simulink model "Speed_Limiter"  (R2022b)
settings: configuration reference "CommonModelConfiguration" (kept outside this file)
undefined symbols (not defined in the file): cc_param_36, LCFG_ActivationDeactivation, LCFG_DSF_Timeout, LCFG_SL_IntStsDelay, LCFG_SL_Tmr1, LCFG_SL_Tmr2
settings Model: Creator=rkallum  LastModifiedBy=OTHOMSO1
settings ConfigSetRef: SourceName=CommonModelConfiguration  SourceLocation=Base Workspace

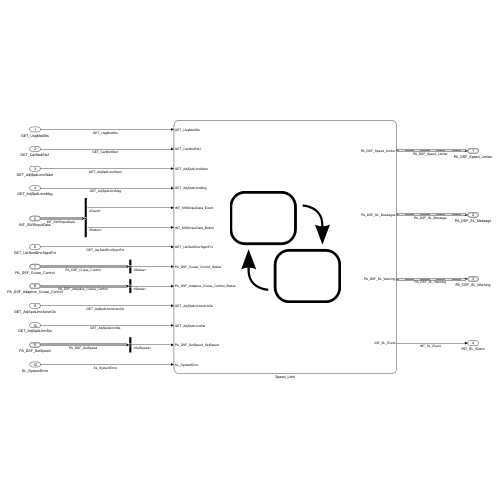
[thumbnail: Simulink's stored preview of the top-level diagram]
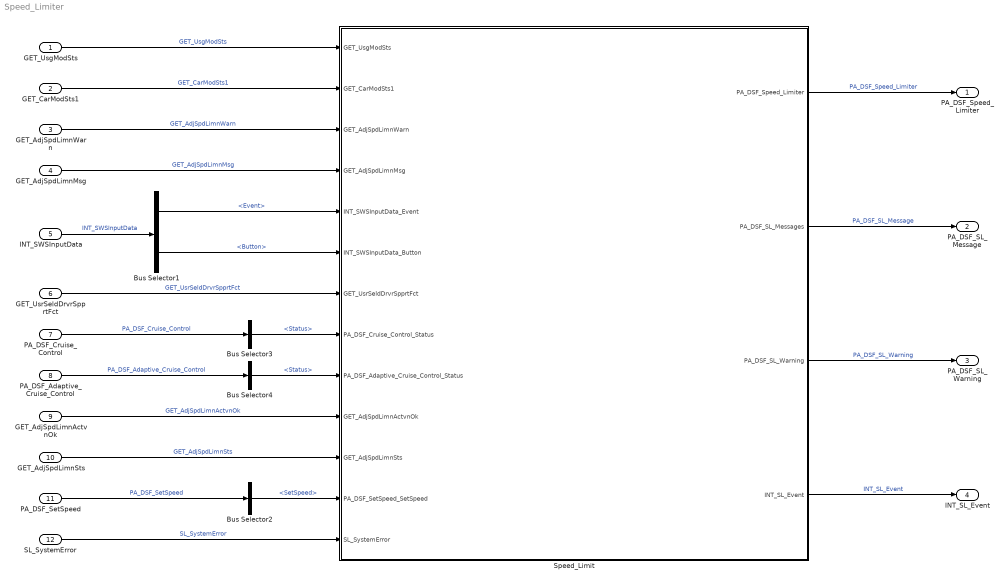
== system Speed_Limiter ==
  GET_UsgModSts : Inport
  GET_CarModSts1 : Inport  Port=2
  GET_AdjSpdLimnWarn : Inport  Port=3
  GET_AdjSpdLimnMsg : Inport  Port=4
  INT_SWSInputData : Inport  Port=5  OutDataTypeStr=Bus: SWSInputData  LockScale=on
  GET_UsrSeldDrvrSpprtFct : Inport  Port=6
  PA_DSF_Cruise_Control : Inport  Port=7  OutDataTypeStr=Bus: PA_DSF
  PA_DSF_Adaptive_Cruise_Control : Inport  Port=8  OutDataTypeStr=Bus: PA_DSF_ACC
  GET_AdjSpdLimnActvnOk : Inport  Port=9
  GET_AdjSpdLimnSts : Inport  Port=10
  PA_DSF_SetSpeed : Inport  Port=11  OutDataTypeStr=Bus: PA_StatusAndValueAndDoubleAndDouble
  SL_SystemError : Inport  Port=12  OutDataTypeStr=boolean
  Bus Selector1 : BusSelector  OutputSignals=Event,Button
  Bus Selector2 : BusSelector  OutputSignals=SetSpeed
  Bus Selector3 : BusSelector  OutputSignals=Status
  Bus Selector4 : BusSelector  OutputSignals=Status
  Speed_Limit : Stateflow chart  TreatAsAtomicUnit=on
  PA_DSF_Speed_Limiter : Outport  OutDataTypeStr=Bus: PA_DSF  VectorParamsAs1DForOutWhenUnconnected=off
  PA_DSF_SL_Message : Outport  Port=2  OutDataTypeStr=Bus: PA_DSF_Message  VectorParamsAs1DForOutWhenUnconnected=off
  PA_DSF_SL_Warning : Outport  Port=3  OutDataTypeStr=Bus: PA_StatusAndOffOnValue  VectorParamsAs1DForOutWhenUnconnected=off
  INT_SL_Event : Outport  Port=4  OutDataTypeStr=Enum: E_DSF_Event  VectorParamsAs1DForOutWhenUnconnected=off
  wires:
  Speed_Limit/1(PA_DSF_Speed_Limiter) -> PA_DSF_Speed_Limiter/1  "PA_DSF_Speed_Limiter"
  Speed_Limit/2(PA_DSF_SL_Messages) -> PA_DSF_SL_Message/1  "PA_DSF_SL_Message"
  Speed_Limit/3(PA_DSF_SL_Warning) -> PA_DSF_SL_Warning/1  "PA_DSF_SL_Warning"
  Speed_Limit/4(INT_SL_Event) -> INT_SL_Event/1  "INT_SL_Event"
  GET_CarModSts1/1 -> Speed_Limit/2(GET_CarModSts1)  "GET_CarModSts1"
  GET_AdjSpdLimnWarn/1 -> Speed_Limit/3(GET_AdjSpdLimnWarn)  "GET_AdjSpdLimnWarn"
  GET_AdjSpdLimnMsg/1 -> Speed_Limit/4(GET_AdjSpdLimnMsg)  "GET_AdjSpdLimnMsg"
  GET_UsrSeldDrvrSpprtFct/1 -> Speed_Limit/7(GET_UsrSeldDrvrSpprtFct)  "GET_UsrSeldDrvrSpprtFct"
  GET_AdjSpdLimnActvnOk/1 -> Speed_Limit/10(GET_AdjSpdLimnActvnOk)  "GET_AdjSpdLimnActvnOk"
  GET_AdjSpdLimnSts/1 -> Speed_Limit/11(GET_AdjSpdLimnSts)  "GET_AdjSpdLimnSts"
  GET_UsgModSts/1 -> Speed_Limit/1(GET_UsgModSts)  "GET_UsgModSts"
  PA_DSF_Cruise_Control/1 -> Bus Selector3/1  "PA_DSF_Cruise_Control"
  PA_DSF_Adaptive_Cruise_Control/1 -> Bus Selector4/1  "PA_DSF_Adaptive_Cruise_Control"
  PA_DSF_SetSpeed/1 -> Bus Selector2/1  "PA_DSF_SetSpeed"
  SL_SystemError/1 -> Speed_Limit/13(SL_SystemError)  "SL_SystemError"
  INT_SWSInputData/1 -> Bus Selector1/1  "INT_SWSInputData"
  Bus Selector1/1 -> Speed_Limit/5(INT_SWSInputData_Event)  "<Event>"
  Bus Selector1/2 -> Speed_Limit/6(INT_SWSInputData_Button)  "<Button>"
  Bus Selector2/1 -> Speed_Limit/12(PA_DSF_SetSpeed_SetSpeed)  "<SetSpeed>"
  Bus Selector3/1 -> Speed_Limit/8(PA_DSF_Cruise_Control_Status)  "<Status>"
  Bus Selector4/1 -> Speed_Limit/9(PA_DSF_Adaptive_Cruise_Control_Status)  "<Status>"

== stateflow chart Speed_Limiter/Speed_Limit ==
  state CARCONFIG_INVALID
    entry:  PA_DSF_Speed_Limiter.Status=E_CommonStatus.NotPresent;
    PA_DSF_SL_Messages.Status=E_CommonStatus.NotPresent;
    PA_DSF_SL_Warning.Status=E_CommonStatus.NotPresent;
    PA_DSF_Speed_Limiter.Value=E_DSF_Value.DSF_Selected;
    PA_DSF_SL_Warning.Value=E_OffOn.Off;
    INT_SL_Event=E_DSF_Event.NoReq;
  state SYSTEM_OK
    state NOT_ACTIVE
      entry: PA_DSF_Speed_Limiter.Status=E_CommonStatus.Disabled;
      PA_DSF_SL_Messages.Status=E_CommonStatus.Disabled;
      PA_DSF_SL_Warning.Status=E_CommonStatus.Disabled;
      PA_DSF_SL_Warning.Value=E_OffOn.Off;
      INT_SL_Event=E_DSF_Event.NoReq;
      state MESSAGES_OFF
        entry:
        PA_DSF_SL_Messages.Value=E_DSF_Messages.Messages_Off;
        PA_DSF_Speed_Limiter.Value=E_DSF_Value.DSF_Selected;
      state CANCEL_WARNING
        entry:
        PA_DSF_SL_Messages.Value=E_DSF_Messages.Messages_CancelWarning;
        PA_DSF_Speed_Limiter.Value=E_DSF_Value.DSF_Selected;
      (default) -> (junction 220)
      (junction 220) -> (junction 224) [order 1] : [PA_DSF_Speed_Limiter.Value==E_DSF_Value.DSF_Active]
      (junction 220) -> MESSAGES_OFF [order 2]
      (junction 224) -> SYSTEM_OK.NOT_ACTIVE.CANCEL_WARNING
      SYSTEM_OK.NOT_ACTIVE.CANCEL_WARNING -> MESSAGES_OFF : [after(LCFG_DSF_Timeout, sec)]
    state PENDING
    state PENDING1
    state ACTIVE
      state WARNING [parallel]
        entry: PA_DSF_SL_Warning.Status=E_CommonStatus.Available;
        settings: executionOrder=1
        state ON
          entry: PA_DSF_SL_Warning.Value=E_OffOn.On;
        state OFF
          entry: PA_DSF_SL_Warning.Value=E_OffOn.Off;
        (default) -> OFF
        OFF -> SYSTEM_OK.ACTIVE.WARNING.ON : [PA_DSF_Speed_Limiter.Value==E_DSF_Value.DSF_Active &&...
            | (GET_AdjSpdLimnWarn==AdjSpdLimnWarnCoding.AdjSpdLimnWarnCoding_VisWarn ||...
            | GET_AdjSpdLimnWarn==AdjSpdLimnWarnCoding.AdjSpdLimnWarnCoding_SoundAndVisWarn)]
        SYSTEM_OK.ACTIVE.WARNING.ON -> OFF : [PA_DSF_Speed_Limiter.Value~=E_DSF_Value.DSF_Active ||...
            | (GET_AdjSpdLimnWarn~=AdjSpdLimnWarnCoding.AdjSpdLimnWarnCoding_VisWarn &&...
            | GET_AdjSpdLimnWarn~=AdjSpdLimnWarnCoding.AdjSpdLimnWarnCoding_SoundAndVisWarn)]
      state MESSAGES [parallel]
        entry: PA_DSF_SL_Messages.Status=E_CommonStatus.Available;
        settings: executionOrder=2
        state retVal = slMessages [function]
          state retVal2 = slActivationReq [function]
            (default) -> (junction 357)
            (junction 357) -> (junction 358) [order 1] : [(GET_AdjSpdLimnSts~=AdjSpdLimnSts2.AdjSpdLimnSts2_Actv)...
                | && (GET_AdjSpdLimnActvnOk == OnOff1.OnOff1_Off)...
                | && (INT_SWSInputData_Button ==  E_SWSButton.BtnL1Req)...
                | && (INT_SWSInputData_Event ==  E_SWSEvent.Push)]
            (junction 357) -> (junction 360) [order 2]
            (junction 358) -> (junction 359)
            (junction 360) -> (junction 359) [order 1] : [(GET_AdjSpdLimnSts~=AdjSpdLimnSts2.AdjSpdLimnSts2_Actv)...
                | && (GET_AdjSpdLimnActvnOk == OnOff1.OnOff1_Off)...
                | && (INT_SWSInputData_Button ==  E_SWSButton.BtnL5Req)...
                | && (INT_SWSInputData_Event ==  E_SWSEvent.Push)...
                | && (PA_DSF_SetSpeed_SetSpeed~=0)]
            (junction 359) -> (junction 361) : {retVal2 = true;}
            (junction 360) -> (junction 362) [order 2] : {retVal2 = false;}
            (junction 361) -> (junction 362)
            (junction 362) -> (junction 363)
          (default) -> (junction 391)
          (junction 391) -> (junction 374) [order 1] : [hasChangedTo(GET_AdjSpdLimnMsg,  AdjSpdLimnMsg1.AdjSpdLimnMsg1_AdjSpdLimnCncl)]
              | {PA_DSF_SL_Messages.Value=E_DSF_Messages.Messages_CancelWarning;}
          (junction 391) -> (junction 392) [order 2]
          (junction 374) -> (junction 375)
          (junction 392) -> (junction 375) [order 1] : [(GET_AdjSpdLimnMsg == AdjSpdLimnMsg1.AdjSpdLimnMsg1_AdjSpdLimnInhb) &&...
              | slActivationReq()]
              | {PA_DSF_SL_Messages.Value=E_DSF_Messages.Messages_Unavailable;}
          (junction 392) -> (junction 399) [order 2] : {retVal = false;}
          (junction 375) -> (junction 400) : {retVal = true;}
          (junction 400) -> (junction 399)
          (junction 399) -> (junction 396)
        state HIDE_MESSAGES
          entry: PA_DSF_SL_Messages.Value = E_DSF_Messages.Messages_Off;
        state SHOW_MESSAGES
        (default) -> HIDE_MESSAGES
        HIDE_MESSAGES -> SHOW_MESSAGES : [slMessages()]
        SHOW_MESSAGES -> HIDE_MESSAGES [order 2] : [after(LCFG_DSF_Timeout,sec) ||...
            | hasChangedTo(GET_AdjSpdLimnSts,AdjSpdLimnSts2.AdjSpdLimnSts2_Actv)]
        SHOW_MESSAGES -> SHOW_MESSAGES [order 1] : [slMessages()]
      state SL [parallel]
        entry: PA_DSF_Speed_Limiter.Status=E_CommonStatus.Available;
        settings: executionOrder=3
        state STANDBY
          entry:
          PA_DSF_Speed_Limiter.Value=E_DSF_Value.DSF_Standby;
          state NO_EVENT
            entry: INT_SL_Event=E_DSF_Event.NoReq
          state EVENT
          (default) -> SYSTEM_OK.ACTIVE.SL.STANDBY.EVENT
          SYSTEM_OK.ACTIVE.SL.STANDBY.EVENT -> SYSTEM_OK.ACTIVE.SL.STANDBY.NO_EVENT : [after(LCFG_ActivationDeactivation,sec)]
        state SELECTED
          entry:
          PA_DSF_Speed_Limiter.Value=E_DSF_Value.DSF_Selected;
        state ON
          entry:
          PA_DSF_Speed_Limiter.Value=E_DSF_Value.DSF_Active;
          state EVENT
          state NO_EVENT
            entry: INT_SL_Event=E_DSF_Event.NoReq
          (default) -> SYSTEM_OK.ACTIVE.SL.ON.EVENT
          SYSTEM_OK.ACTIVE.SL.ON.EVENT -> SYSTEM_OK.ACTIVE.SL.ON.NO_EVENT : [after(LCFG_ActivationDeactivation,sec)]
        (default) -> SELECTED
        SELECTED -> SYSTEM_OK.ACTIVE.SL.ON [order 1] : [(INT_SWSInputData_Button==E_SWSButton.BtnL1Req &&...
            | hasChangedTo(INT_SWSInputData_Event, E_SWSEvent.Push) &&...
            | GET_AdjSpdLimnActvnOk==OnOff1.OnOff1_On)]
            | {INT_SL_Event=E_DSF_Event.Activation;}
        SELECTED -> SYSTEM_OK.ACTIVE.SL.ON [order 2] : [after(LCFG_SL_IntStsDelay, sec) &&...
            | (GET_AdjSpdLimnSts==AdjSpdLimnSts2_Actv ||...
            | GET_AdjSpdLimnSts==AdjSpdLimnSts2_Ovrd)]
        STANDBY -> SYSTEM_OK.ACTIVE.SL.ON [order 1] : [(INT_SWSInputData_Button==E_SWSButton.BtnL1Req &&...
            | hasChangedTo(INT_SWSInputData_Event, E_SWSEvent.Push) &&...
            | GET_AdjSpdLimnActvnOk==OnOff1.OnOff1_On) &&...
            | INT_SL_Event==E_DSF_Event.NoReq]
            | {INT_SL_Event=E_DSF_Event.Activation;}
        STANDBY -> SYSTEM_OK.ACTIVE.SL.ON [order 3] : [(after(LCFG_SL_IntStsDelay, sec) &&...
            | (GET_AdjSpdLimnSts==AdjSpdLimnSts2_Actv ||...
            | GET_AdjSpdLimnSts==AdjSpdLimnSts2_Ovrd))]
        STANDBY -> SYSTEM_OK.ACTIVE.SL.ON [order 2] : [INT_SWSInputData_Button==E_SWSButton.BtnL5Req &&...
            | hasChangedTo(INT_SWSInputData_Event, E_SWSEvent.Push) &&...
            | GET_AdjSpdLimnActvnOk==OnOff1.OnOff1_On &&...
            | PA_DSF_SetSpeed_SetSpeed~=0 &&...
            | INT_SL_Event==E_DSF_Event.NoReq]
            | {INT_SL_Event=E_DSF_Event.Resume;}
        SYSTEM_OK.ACTIVE.SL.ON -> STANDBY [order 1] : [(INT_SWSInputData_Button==E_SWSButton.BtnL1Req &&...
            | hasChangedTo(INT_SWSInputData_Event, E_SWSEvent.Push) &&...
            | INT_SL_Event==E_DSF_Event.NoReq) ||...
            | INT_SWSInputData_Event == E_SWSEvent.Deactivation]
            | {INT_SL_Event=E_DSF_Event.Deactivation;}
        SYSTEM_OK.ACTIVE.SL.ON -> STANDBY [order 2] : [(after(LCFG_SL_IntStsDelay, sec) &&...
            | (GET_AdjSpdLimnSts~=AdjSpdLimnSts2_Actv &&...
            | GET_AdjSpdLimnSts~=AdjSpdLimnSts2_Ovrd))]
    state isActive = ActivationCheck [function]
      (default) -> (junction 37)
      (junction 37) -> (junction 38) [order 1] : [GET_CarModSts1 == CarModSts1.CarModSts1_CarModNorm &&...
          | GET_UsgModSts == UsgModSts1.UsgModSts1_UsgModDrvg &&...
          | (GET_UsrSeldDrvrSpprtFct==DrvrSpprtFct.DrvrSpprtFct_SL ||...
          | PA_DSF_Speed_Limiter.Value==E_DSF_Value.DSF_Active) &&...
          | PA_DSF_Cruise_Control_Status~=E_CommonStatus.Available &&...
          | PA_DSF_Adaptive_Cruise_Control_Status~=E_CommonStatus.Available]
      (junction 37) -> (junction 40) [order 2] : {isActive=false;}
      (junction 38) -> (junction 39) : {isActive=true;}
      (junction 39) -> (junction 40)
      (junction 40) -> (junction 41)
    (default) -> NOT_ACTIVE
    NOT_ACTIVE -> PENDING : [ActivationCheck()]
    PENDING -> NOT_ACTIVE [order 2] : [~ActivationCheck()]
    PENDING1 -> NOT_ACTIVE [order 1] : [~ActivationCheck() &&...
        | after(LCFG_SL_Tmr1,sec)]
    PENDING -> ACTIVE [order 1] : [ActivationCheck() &&...
        | after(LCFG_SL_Tmr2,sec)]
    PENDING1 -> ACTIVE [order 2] : [ActivationCheck()]
    ACTIVE -> PENDING1 : [~ActivationCheck()]
  state SYSTEM_ERROR
    entry:
    PA_DSF_Speed_Limiter.Status=E_CommonStatus.SystemError;
    PA_DSF_SL_Messages.Status=E_CommonStatus.SystemError;
    PA_DSF_SL_Warning.Status=E_CommonStatus.SystemError;
    PA_DSF_SL_Warning.Value=E_OffOn.Off;
    INT_SL_Event=E_DSF_Event.NoReq;
    state retVal = slActivationReq [function]
      (default) -> (junction 228)
      (junction 228) -> (junction 229) [order 1] : [(INT_SWSInputData_Button==E_SWSButton.BtnL1Req ||...
          | INT_SWSInputData_Button==E_SWSButton.BtnL5Req) &&...
          | hasChangedTo(INT_SWSInputData_Event, E_SWSEvent.Push) &&...
          | GET_UsrSeldDrvrSpprtFct==DrvrSpprtFct.DrvrSpprtFct_SL]
      (junction 228) -> (junction 230) [order 2] : {retVal=false;}
      (junction 229) -> (junction 231) : {retVal=true;}
      (junction 231) -> (junction 230)
      (junction 230) -> (junction 232)
    state CANCEL_WARNING
      entry:
      PA_DSF_SL_Messages.Value=E_DSF_Messages.Messages_CancelWarning;
      PA_DSF_Speed_Limiter.Value=E_DSF_Value.DSF_Selected;
    state UNAVAILABLE
      entry:
      PA_DSF_SL_Messages.Value=E_DSF_Messages.Messages_Unavailable;
    state NO_MESSAGES
      entry:
      PA_DSF_SL_Messages.Value=E_DSF_Messages.Messages_Off;
      PA_DSF_Speed_Limiter.Value=E_DSF_Value.DSF_Selected;
    (default) -> (junction 252)
    (junction 252) -> (junction 245) [order 1] : [PA_DSF_Speed_Limiter.Value==E_DSF_Value.DSF_Active]
    (junction 252) -> NO_MESSAGES [order 2]
    (junction 245) -> SYSTEM_ERROR.CANCEL_WARNING
    UNAVAILABLE -> UNAVAILABLE [order 2] : [slActivationReq()]
    SYSTEM_ERROR.CANCEL_WARNING -> UNAVAILABLE [order 2] : [slActivationReq()]
    UNAVAILABLE -> NO_MESSAGES [order 1] : [after(LCFG_DSF_Timeout, sec)]
    NO_MESSAGES -> UNAVAILABLE : [slActivationReq()]
    SYSTEM_ERROR.CANCEL_WARNING -> NO_MESSAGES [order 1] : [after(LCFG_DSF_Timeout, sec)]
  (default) -> (junction 196)
  (junction 196) -> CARCONFIG_INVALID [order 2]
  (junction 196) -> (junction 205) [order 1] : [cc_param_36>1]
  (junction 205) -> SYSTEM_OK [order 2]
  (junction 205) -> (junction 206) [order 1] : [SL_SystemError==true ||...
      | INT_SWSInputData_Event==E_SWSEvent.ButtonStuck]
  SYSTEM_OK -> SYSTEM_ERROR : [SL_SystemError==true ||...
      | INT_SWSInputData_Event==E_SWSEvent.ButtonStuck]
  SYSTEM_ERROR -> SYSTEM_OK : [SL_SystemError==false &&...
      | INT_SWSInputData_Event~=E_SWSEvent.ButtonStuck]
  (junction 206) -> SYSTEM_ERROR
  data: retVal2 function_output; retVal function_output; isActive function_output boolean; retVal function_output; PA_DSF_Speed_Limiter output Bus: PA_DSF =0; GET_UsgModSts input Enum: UsgModSts1; GET_CarModSts1 input Enum: CarModSts1; GET_AdjSpdLimnWarn input Enum: AdjSpdLimnWarnCoding; GET_AdjSpdLimnMsg input Enum: AdjSpdLimnMsg1; INT_SWSInputData_Event input Enum: E_SWSEvent; INT_SWSInputData_Button input Enum: E_SWSButton; PA_DSF_SL_Messages output Bus: PA_DSF_Message =0; PA_DSF_SL_Warning output Bus: PA_StatusAndOffOnValue =0; LCFG_DSF_Timeout parameter; LCFG_SL_Tmr1 parameter; LCFG_SL_Tmr2 parameter; cc_param_36 parameter; GET_UsrSeldDrvrSpprtFct input Enum: DrvrSpprtFct; PA_DSF_Cruise_Control_Status input Enum: E_CommonStatus; PA_DSF_Adaptive_Cruise_Control_Status input Enum: E_CommonStatus; INT_SL_Event output Enum: E_DSF_Event; GET_AdjSpdLimnActvnOk input Enum: OnOff1; GET_AdjSpdLimnSts input Enum: AdjSpdLimnSts2; PA_DSF_SetSpeed_SetSpeed input double; LCFG_SL_IntStsDelay parameter; SL_SystemError input boolean; LCFG_ActivationDeactivation parameter double
